simulink model "sine_gen_v1"  (R2025a)
settings: Solver=VariableStepAuto  StartTime=0.0  StopTime=2e-4  RelTol=1e-3
model workspace (MAT data in the model file):
  NoaFutureIOMap{1}.PortName = 'amp'
  NoaFutureIOMap{1}.PortType = 'Inport'
  NoaFutureIOMap{1}.DataType = 'sfix32_En21'
  NoaFutureIOMap{1}.IOInterface = 'AXI4-Lite'
  NoaFutureIOMap{1}.IOInterfaceMapping = 'x"100"'
  NoaFutureIOMap{2}.PortName = 'freq'
  NoaFutureIOMap{2}.PortType = 'Inport'
  NoaFutureIOMap{2}.DataType = 'uint32'
  NoaFutureIOMap{2}.IOInterface = 'AXI4-Lite'
  NoaFutureIOMap{2}.IOInterfaceMapping = 'x"104"'
  NoaFutureIOMap{3}.PortName = 'sine'
  NoaFutureIOMap{3}.PortType = 'Outport'
  NoaFutureIOMap{3}.DataType = 'sfix32_En21'
  NoaFutureIOMap{3}.IOInterface = 'DAQ Channel 0 [0:31]'
  NoaFutureIOMap{3}.IOInterfaceMapping = '[0:31]'
  NoaFutureIOMap{4}.PortName = 'sine_analog'
  NoaFutureIOMap{4}.PortType = 'Outport'
  NoaFutureIOMap{4}.DataType = 'sfix32_En23'
  NoaFutureIOMap{4}.IOInterface = 'Analog Output 0 [0:31]'
  NoaFutureIOMap{4}.IOInterfaceMapping = '[0:31]'
  NoaFutureIOMap{4}.NoaBlockParameters.SignalMin = '-300'
  NoaFutureIOMap{4}.NoaBlockParameters.SignalMax = '300'
  NoaFutureIOMap{4}.NoaBlockParameters.VoltageMin = '-3'
  NoaFutureIOMap{4}.NoaBlockParameters.VoltageMax = '3'
  NoaFutureIOMap{4}.NoaBlockParameters.LUT_Signals = '[-300 -240 -180 -120  -60    0   60  120  180  240  300]'
  NoaFutureIOMap{4}.NoaBlockParameters.LUT_Values = '[-3        -2.4        -1.8        -1.2        -0.6           0         0.6         1.2         1.8         2.4           3]'
undefined symbols (not defined in the file): period
libraries: hdlsllib x2, library_AnalogOut x1
settings Model: Creator=tarko  LastModifiedBy=ambre
settings OptimizationCC: BlockReduction=off  ConditionallyExecuteInputs=off  DefaultParameterBehavior=Inlined
settings DebuggingCC: AlgebraicLoopMsg=error
settings HardwareCC: ProdBitPerPointer=32.0  ProdBitPerSizeT=32.0  ProdBitPerPtrDiffT=32.0  ProdLargestAtomicFloat=None  ProdIntDivRoundTo=Undefined  ProdEndianess=Unspecified  ProdWordSize=32.0  ProdHWDeviceType=ASIC/FPGA->ASIC/FPGA  TargetBitPerPointer=64.0  TargetBitPerSizeT=64.0  TargetBitPerPtrDiffT=64.0  TargetLongLongMode=on  TargetIntDivRoundTo=Zero  TargetEndianess=LittleEndian  TargetWordSize=64.0  TargetHWDeviceType=Custom Processor->MATLAB Host Computer  ProdEqTarget=off

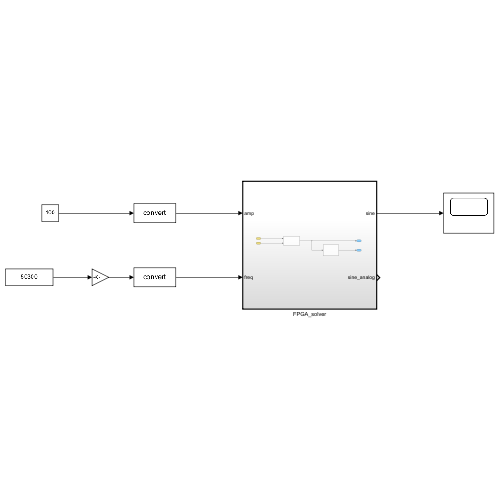
[thumbnail: Simulink's stored preview of the top-level diagram]
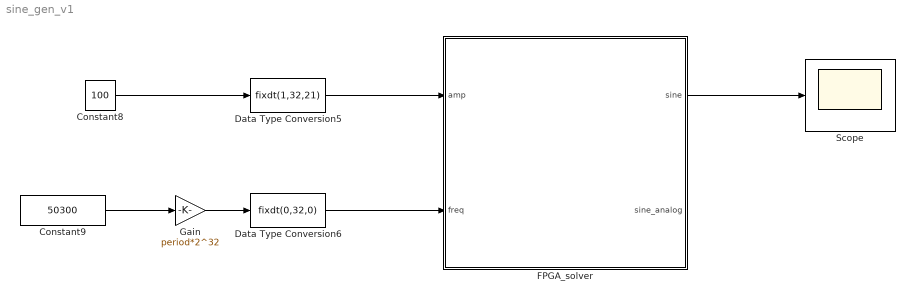
== system sine_gen_v1 ==
  Constant8 : Constant  Value=100  SampleTime=period
  Constant9 : Constant  Value=50300  SampleTime=period
  Data Type Conversion5 : DataTypeConversion  OutDataTypeStr=fixdt(1,32,21)  SaturateOnIntegerOverflow=off  RndMeth=Floor
  Data Type Conversion6 : DataTypeConversion  OutDataTypeStr=fixdt(0,32,0)  SaturateOnIntegerOverflow=off  RndMeth=Floor
  FPGA_solver : Subsystem  TreatAsAtomicUnit=on
  Gain : Gain  Gain=period*2^32
  Scope : Scope
      settings: ActiveDisplayYMinimum=-125  ActiveDisplayYMaximum=125
  wires:
  Constant8/1 -> Data Type Conversion5/1
  Constant9/1 -> Gain/1
  Gain/1 -> Data Type Conversion6/1
  Data Type Conversion5/1 -> FPGA_solver/1(amp)
  Data Type Conversion6/1 -> FPGA_solver/2(freq)
  FPGA_solver/1(sine) -> Scope/1

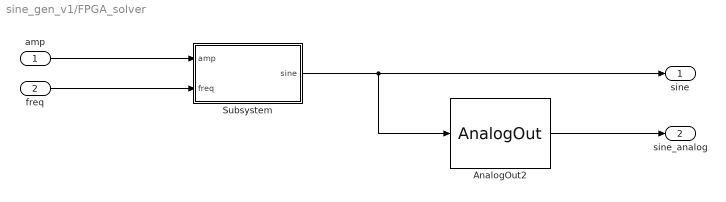
== system sine_gen_v1/FPGA_solver ==
  amp : Inport
  freq : Inport  Port=2
  AnalogOut2 : library_AnalogOut/AnalogOut  SignalMin=-300  SignalMax=300  VoltageMin=-3  VoltageMax=3
  Subsystem : Subsystem
  sine : Outport
  sine_analog : Outport  Port=2
  wires:
  Subsystem/1(sine) -> AnalogOut2/1, sine/1
  amp/1 -> Subsystem/1(amp)
  freq/1 -> Subsystem/2(freq)
  AnalogOut2/1 -> sine_analog/1

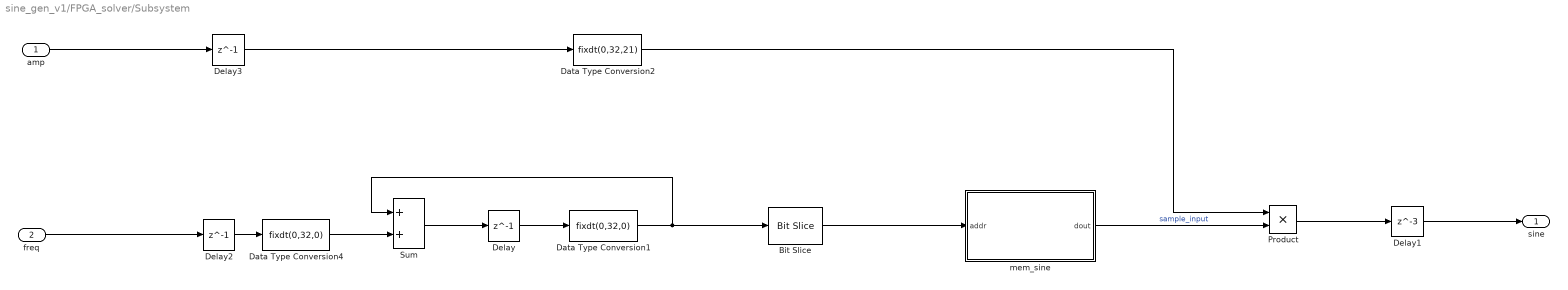
== system sine_gen_v1/FPGA_solver/Subsystem ==
  amp : Inport
  freq : Inport  Port=2
  Bit Slice : hdlsllib/Logic and Bit Operations/Bit Slice  lidx=31  ridx=22
  Data Type Conversion1 : DataTypeConversion  OutDataTypeStr=fixdt(0,32,0)  SaturateOnIntegerOverflow=off  RndMeth=Floor
  Data Type Conversion2 : DataTypeConversion  OutDataTypeStr=fixdt(0,32,21)  SaturateOnIntegerOverflow=off  RndMeth=Floor
  Data Type Conversion4 : DataTypeConversion  OutDataTypeStr=fixdt(0,32,0)  SaturateOnIntegerOverflow=off  RndMeth=Floor
  Delay : Delay  DelayLength=1  InitialCondition=0
  Delay1 : Delay  DelayLength=3  InitialCondition=0
  Delay2 : Delay  DelayLength=1  InitialCondition=(50300*period)*2^32
  Delay3 : Delay  DelayLength=1  InitialCondition=100
  Product : Product  OutDataTypeStr=fixdt(1,32,21)
  Sum : Sum  OutDataTypeStr=uint32
  mem_sine : Subsystem  mask{data=sin(2*pi*(0:1023)/1024), bw=32}
      mask prompts: data "Initial Data"; bw "Bitwidth"
  sine : Outport
  wires:
  freq/1 -> Delay2/1
  Data Type Conversion2/1 -> Product/1
  Delay/1 -> Data Type Conversion1/1
  Data Type Conversion1/1 -> Sum/1, Bit Slice/1
  Data Type Conversion4/1 -> Sum/2
  Delay3/1 -> Data Type Conversion2/1
  Bit Slice/1 -> mem_sine/1(addr)
  mem_sine/1(dout) -> Product/2  "sample_input"
  Sum/1 -> Delay/1
  Delay2/1 -> Data Type Conversion4/1
  Product/1 -> Delay1/1
  amp/1 -> Delay3/1
  Delay1/1 -> sine/1

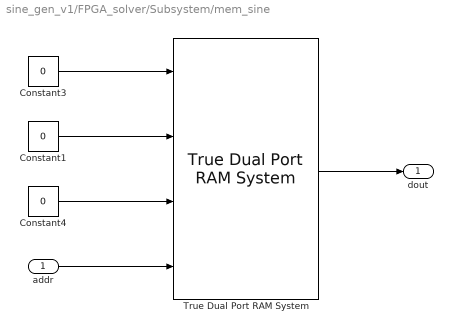
== system sine_gen_v1/FPGA_solver/Subsystem/mem_sine ==
  addr : Inport
  Constant1 : Constant  Value=0  OutDataTypeStr=fixdt(0,10,0)  SampleTime=period
  Constant3 : Constant  Value=0  OutDataTypeStr=fixdt(1,bw,21)  SampleTime=period
  Constant4 : Constant  Value=0  OutDataTypeStr=boolean  SampleTime=period
  True Dual Port RAM System : hdlsllib/HDL RAMs/True Dual Port RAM System  RAMType=Simple dual port  AsyncRead=off  WriteOutputValue=Old data  RAMInitialValue=data  allowBusInputs=off  WritesHaveOutput=on  NumReads=0  NumWrites=1  SimulateUsing=Code generation  ModelRAMDelay=on  VectorAccess=Parallel
  dout : Outport
  wires:
  True Dual Port RAM System/1 -> dout/1
  Constant1/1 -> True Dual Port RAM System/2
  Constant3/1 -> True Dual Port RAM System/1
  Constant4/1 -> True Dual Port RAM System/3
  addr/1 -> True Dual Port RAM System/4
